simulink library "actuator_processing_lib"  (R2018b)
settings: Solver=VariableStepAuto  StartTime=0.0  StopTime=10.0  RelTol=1e-3
settings Model: Creator=colem  LastModifiedBy=colem

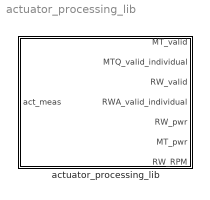
== system actuator_processing_lib ==
  actuator_processing_lib : Subsystem

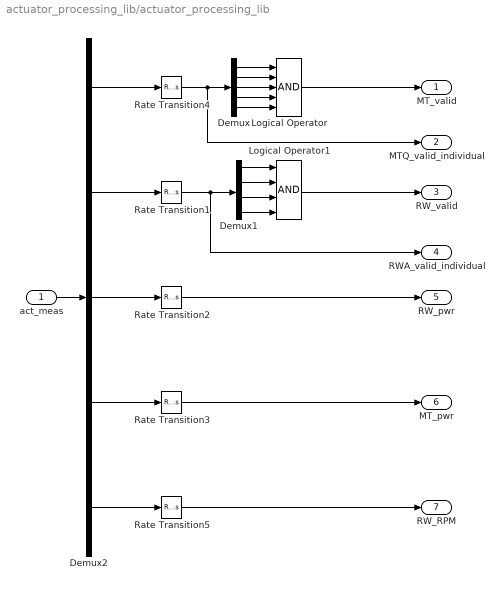
== system actuator_processing_lib/actuator_processing_lib ==
  act_meas : Inport
  Demux : Demux  Outputs=[1 1 1 1 1]
  Demux1 : Demux  Outputs=[1 1 1 1]
  Demux2 : Demux  Outputs=[5 4 1 1 4]
  Logical Operator : Logic  Inputs=5  AllPortsSameDT=off  OutDataTypeStr=boolean
  Logical Operator1 : Logic  Inputs=4  AllPortsSameDT=off  OutDataTypeStr=boolean
  Rate Transition{1..5} (5 alike) : RateTransition  OutPortSampleTime=fswParams.sample_time_s
  MT_valid : Outport
  MTQ_valid_individual : Outport  Port=2
  RW_valid : Outport  Port=3
  RWA_valid_individual : Outport  Port=4
  RW_pwr : Outport  Port=5
  MT_pwr : Outport  Port=6
  RW_RPM : Outport  Port=7
  wires:
  Logical Operator1/1 -> RW_valid/1
  Rate Transition1/1 -> RWA_valid_individual/1, Demux1/1
  Demux1/2 -> Logical Operator1/2
  Demux1/1 -> Logical Operator1/1
  Demux1/3 -> Logical Operator1/3
  Demux2/5 -> Rate Transition5/1
  Demux2/4 -> Rate Transition3/1
  Demux2/2 -> Rate Transition1/1
  Demux2/1 -> Rate Transition4/1
  act_meas/1 -> Demux2/1
  Rate Transition4/1 -> MTQ_valid_individual/1, Demux/1
  Rate Transition2/1 -> RW_pwr/1
  Demux2/3 -> Rate Transition2/1
  Rate Transition3/1 -> MT_pwr/1
  Rate Transition5/1 -> RW_RPM/1
  Demux/2 -> Logical Operator/2
  Demux/1 -> Logical Operator/1
  Demux/3 -> Logical Operator/3
  Logical Operator/1 -> MT_valid/1
  Demux/4 -> Logical Operator/4
  Demux/5 -> Logical Operator/5
  Demux1/4 -> Logical Operator1/4
